simulink model "sf_tlbefore"  (Simulink 6.0)
settings: Solver=ode45  StartTime=0.0  StopTime=20  MaxStep=.01  RelTol=1e-3
settings Model: CovMetricSettings=dcmtr  Creator=The MathWorks Inc.  LastModifiedBy=batserve  ExtModeAutoUpdateStatusClock=off
settings OptimizationCC: BooleanDataType=off
settings DebuggingCC: CheckExecutionContextPreStartOutputMsg=on  CheckExecutionContextRuntimeOutputMsg=on  SolverPrmCheckMsg=none
settings HardwareCC: TargetUnknown=on

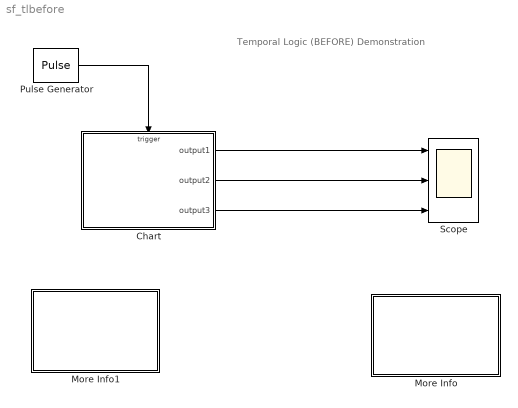
== system sf_tlbefore ==
  note: Temporal Logic (BEFORE) Demonstration
  Chart : Stateflow chart  TreatAsAtomicUnit=on  PropExecContextAcrossSSBoundary=on
  More Info : Subsystem  PropExecContextAcrossSSBoundary=on
      mask Display: disp('Double click\nhere for\ninformation on\nthis demonstration')
  More Info1 : Subsystem  PropExecContextAcrossSSBoundary=on
      settings: OpenFcn=simcad(bdroot);
      mask Display: disp('Double click\nhere for\nSimulink\Stateflow\n Help')
  Pulse Generator : DiscretePulseGenerator  PulseType=Time based  Period=1  PulseWidth=50
  Scope : Scope  NumInputPorts=3
      settings: TimeRange=20  YMin=0~0~-1  YMax=1.25~1.25~1
  wires:
  Pulse Generator/1 -> Chart/Trigger
  Chart/1(output1) -> Scope/1
  Chart/2(output2) -> Scope/2
  Chart/3(output3) -> Scope/3

== system sf_tlbefore/More Info ==
  note: Temporal Logic using the BEFORE function
  note: The BEFORE function allows you to execute a transition or an action before a certain number
      | of events occur. In this example, we illustrate the use of the BEFORE function for three different
      | conditions with three different constraints.
      |
      | In superstate One, two conditions need to be met for the transition out of A_state: signal_one has
      | to be less than 5 before 10 events occur. Since both these conditions are met, the output is set to
      | 1 (after all three parallel states are initialized).
      |
      | In superstate Two, two different conditions need to be met for the transition out of B_state:
      | signal_two has to be less greater than 10 before 20 events occur. These conditions are met later
      | on in the simulation, when signal_two becomes greater than 10.
      |
      | Finally, in superstate Three, two other conditions need to be met for the transition out of C_state:
      | signal_three has to be greater than 11 before 10 events occur. Since this never occurs, output3 is
      | is never set to 1 and thus remains 0 for whole simulation.

== system sf_tlbefore/More Info1 ==

== stateflow chart Chart ==
  state One [parallel]
    state A_state
      on count:signal_one++;
    A_state -> (junction 9) : before(10,count)[signal_one<5]{output1=1;}
    (junction 9) -> A_state
  state Two [parallel]
    state B_state
      on count:signal_two++;
    (junction 10) -> B_state
    B_state -> (junction 10) : before(20,count)[signal_two>10]{output2=1;}
  state Three [parallel]
    state C_state
      on count:signal_three++;
    C_state -> (junction 11) : before(10,count)[signal_three>11]{output3=1;}
    (junction 11) -> C_state
  (default) -> A_state : {signal_one=0;signal_two=0;signal_three=0;}
  data: output1 output double; signal_three local double; output2 output double; output3 output double; signal_one local double; signal_two local double
  events: count input RISING_EDGE_EVENT
